simulink model "controller_2_1_2_3"  (R2024b)
settings: Solver=VariableStepAuto  StartTime=0.0  StopTime=10.0  RelTol=1e-3
undefined symbols (not defined in the file): K, Nu, Nx, rpm2rads, u_bar_max
settings Model: Creator=Enrico  LastModifiedBy=Enrico

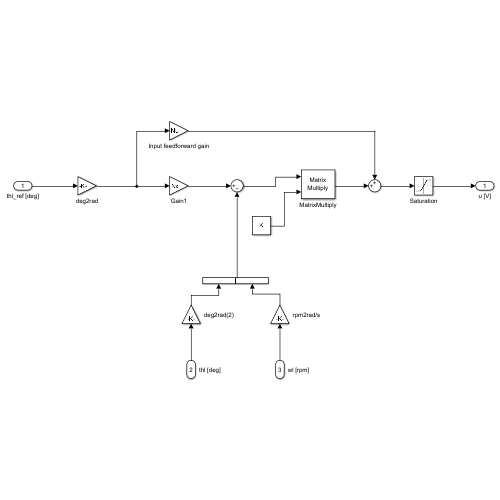
[thumbnail: Simulink's stored preview of the top-level diagram]
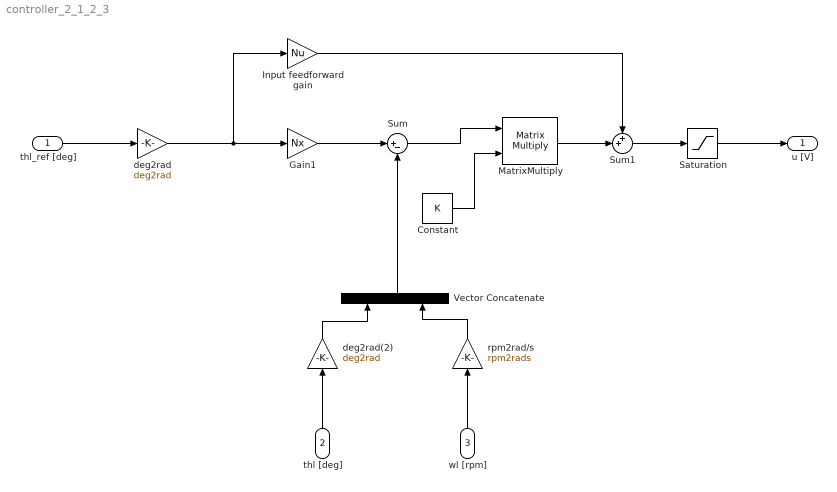
== system controller_2_1_2_3 ==
  thl_ref [deg] : Inport
  thl [deg] : Inport  Port=2
  wl [rpm] : Inport  Port=3
  Constant : Constant  Value=K
  Gain1 : Gain  Gain=Nx
  Input feedforward gain : Gain  Gain=Nu
  MatrixMultiply : Product  Multiplication=Matrix(*)
  Saturation : Saturate  UpperLimit=u_bar_max  LowerLimit=-u_bar_max
  Sum : Sum  Inputs=|+-
  Sum1 : Sum  Inputs=++|
  Vector Concatenate : Concatenate
  deg2rad : Gain  Gain=deg2rad
  deg2rad(2) : Gain  Gain=deg2rad
  rpm2rad/s : Gain  Gain=rpm2rads
  u [V] : Outport
  wires:
  Sum/1 -> MatrixMultiply/1
  Vector Concatenate/1 -> Sum/2
  Input feedforward gain/1 -> Sum1/1
  thl_ref [deg]/1 -> deg2rad/1
  wl [rpm]/1 -> rpm2rad/s/1
  rpm2rad/s/1 -> Vector Concatenate/2
  Constant/1 -> MatrixMultiply/2
  Saturation/1 -> u [V]/1
  Sum1/1 -> Saturation/1
  thl [deg]/1 -> deg2rad(2)/1
  MatrixMultiply/1 -> Sum1/2
  deg2rad/1 -> Input feedforward gain/1, Gain1/1
  Gain1/1 -> Sum/1
  deg2rad(2)/1 -> Vector Concatenate/1
